simulink model "closed_loop"  (R2014a)
settings: Solver=ode3  StartTime=0.0  StopTime=2  FixedStep=0.01  RelTol=1e-3
libraries: simulink x2
settings Model: Creator=Maciek  LastModifiedBy=Maciek

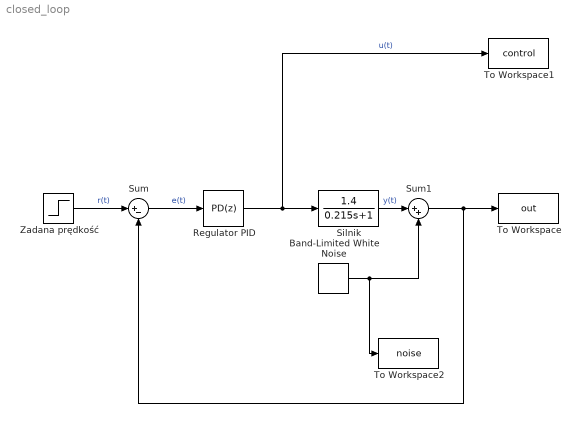
== system closed_loop ==
  Band-Limited White Noise : simulink/Sources/Band-Limited White Noise  Cov=[0.1]  Ts=0.01  seed=[23341]
  Regulator PID : simulink/Continuous/PID Controller  Controller=PD  TimeDomain=Discrete-time  SampleTime=0.01  IntegratorMethod=Forward Euler  FilterMethod=Forward Euler  Form=Parallel  P=6.68696650375987  I=11.6  D=0.0363988255026228  N=52.5630622577478  InitialConditionSource=internal  InitialConditionForIntegrator=0  InitialConditionForFilter=0  ExternalReset=none  LimitOutput=on  UpperSaturationLimit=100  LowerSaturationLimit=-100  LinearizeAsGain=off  AntiWindupMode=clamping  Kb=1  TrackingMode=off  Kt=1  PParamMin=[]  PParamMax=[]  IParamMin=[]  IParamMax=[]  DParamMin=[]  DParamMax=[]  NParamMin=[]  NParamMax=[]  KbParamMin=[]  KbParamMax=[]  KtParamMin=[]  KtParamMax=[]  POutMin=[]  POutMax=[]  IOutMin=[]  IOutMax=[]  DOutMin=[]  DOutMax=[]  NOutMin=[]  NOutMax=[]  KbOutMin=[]  KbOutMax=[]  KtOutMin=[]  KtOutMax=[]  IntegratorOutMin=[]  IntegratorOutMax=[]  FilterOutMin=[]  FilterOutMax=[]  SumOutMin=[]  SumOutMax=[]  SumI1OutMin=[]  SumI1OutMax=[]  SumI2OutMin=[]  SumI2OutMax=[]  SumI3OutMin=[]  SumI3OutMax=[]  SumDOutMin=[]  SumDOutMax=[]  SaturationOutMin=[]  SaturationOutMax=[]  IntegratorContinuousStateAttributes=''  IntegratorStateMustResolveToSignalObject=off  IntegratorRTWStateStorageClass=Auto  FilterContinuousStateAttributes=''  FilterStateMustResolveToSignalObject=off  FilterRTWStateStorageClass=Auto
  Silnik : TransferFcn  Numerator=[1.4]  Denominator=[0.215 1]
  Sum : Sum  Inputs=|+-
  Sum1 : Sum  Inputs=|++
  To Workspace : ToWorkspace  VariableName=out  SaveFormat=Timeseries  SampleTime=-1
  To Workspace1 : ToWorkspace  VariableName=control  SaveFormat=Timeseries  SampleTime=-1
  To Workspace2 : ToWorkspace  VariableName=noise  SaveFormat=Timeseries  SampleTime=-1
  Zadana prędkość : Step  Time=0.01  After=40  SampleTime=0.01
  wires:
  Zadana prędkość/1 -> Sum/1  "r(t)"
  Sum/1 -> Regulator PID/1  "e(t)"
  Regulator PID/1 -> To Workspace1/1, Silnik/1  "u(t)"
  Silnik/1 -> Sum1/1  "y(t)"
  Band-Limited White Noise/1 -> To Workspace2/1, Sum1/2
  Sum1/1 -> Sum/2, To Workspace/1
